simulink model "exp1"  (R2025b)
settings: Solver=VariableStepAuto  StartTime=0.0  StopTime=10.0  RelTol=1e-3
libraries: simulink x1
settings Model: Creator=SUBHASH  LastModifiedBy=SUBHASH

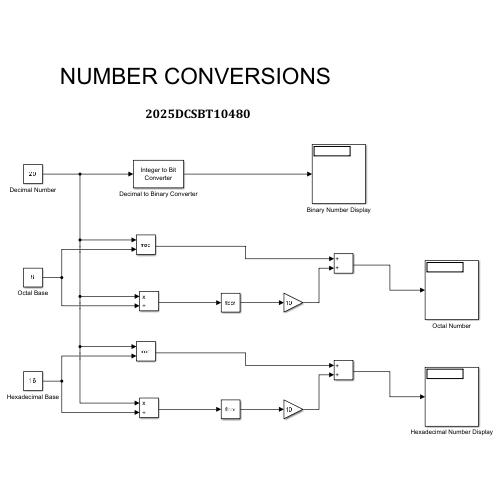
[thumbnail: Simulink's stored preview of the top-level diagram]
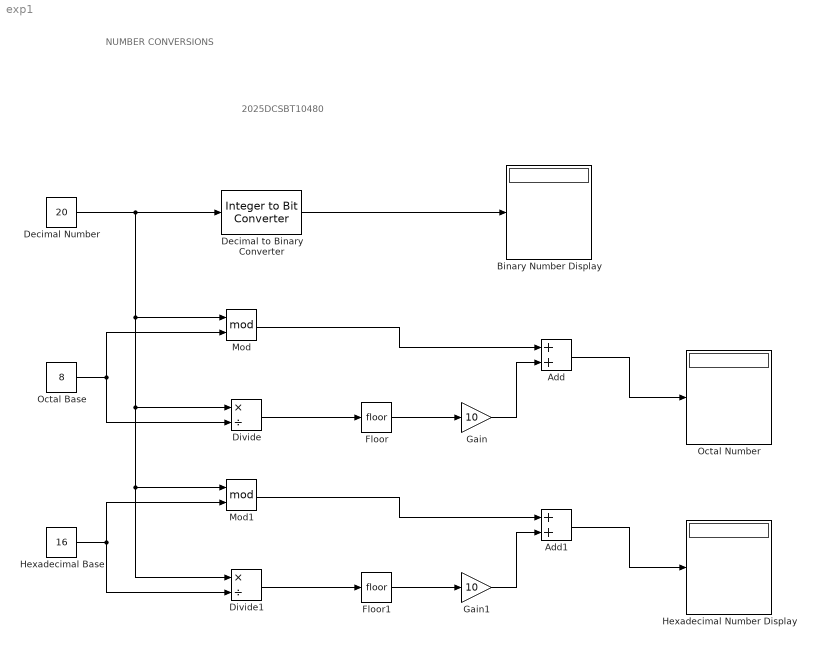
== system exp1 ==
  note: NUMBER CONVERSIONS
  note: 2025DCSBT10480
  Add : Sum
  Add1 : Sum
  Binary Number Display : Display
  Decimal Number : Constant  Value=20
  Decimal to Binary Converter : simulink/Logic and Bit Operations/Integer to Bit Converter  nbits=5  signedInputValues=Unsigned  bitOrder=MSB first  outDtype=Inherit via internal rule
  Divide : Product  Inputs=*/
  Divide1 : Product  Inputs=*/
  Floor : Rounding
  Floor1 : Rounding
  Gain : Gain  Gain=10
  Gain1 : Gain  Gain=10
  Hexadecimal Base : Constant  Value=16
  Hexadecimal Number Display : Display
  Mod : Math  Operator=mod  SignedPower=on
  Mod1 : Math  Operator=mod  SignedPower=on
  Octal Base : Constant  Value=8
  Octal Number : Display
  wires:
  Decimal Number/1 -> Divide1/1, Mod1/1, Divide/1, Mod/1, Decimal to Binary Converter/1
  Decimal to Binary Converter/1 -> Binary Number Display/1
  Octal Base/1 -> Divide/2, Mod/2
  Divide/1 -> Floor/1
  Floor/1 -> Gain/1
  Mod/1 -> Add/1
  Gain/1 -> Add/2
  Add/1 -> Octal Number/1
  Gain1/1 -> Add1/2
  Floor1/1 -> Gain1/1
  Mod1/1 -> Add1/1
  Add1/1 -> Hexadecimal Number Display/1
  Divide1/1 -> Floor1/1
  Hexadecimal Base/1 -> Divide1/2, Mod1/2
